simulink model "sstdr_basic"  (R2024b)
settings: Solver=FixedStepDiscrete  StartTime=0.0  StopTime=0.0005  FixedStep=5e-9  RelTol=1e-3
libraries: spsGroundLib x5, spsSeriesRLCBranchLib x4, spsIdealSwitchLib x3, spsVoltageMeasurementLib x3, spsControlledVoltageSourceLib x1, dspstat3 x1, spsDistributedParametersLineFrequencyDependentLib x1, sps_lib x1
settings Model: Creator=nathanielfargo  LastModifiedBy=nathanielfargo

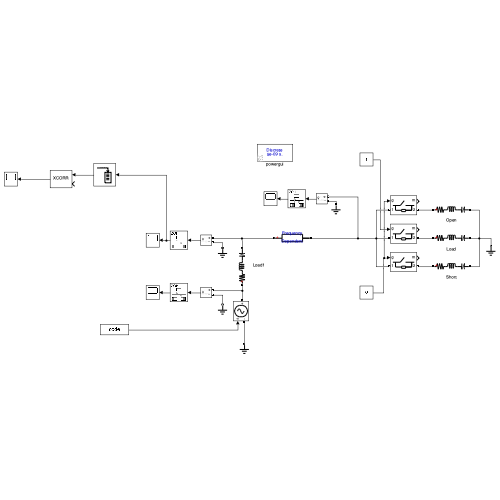
[thumbnail: Simulink's stored preview of the top-level diagram]
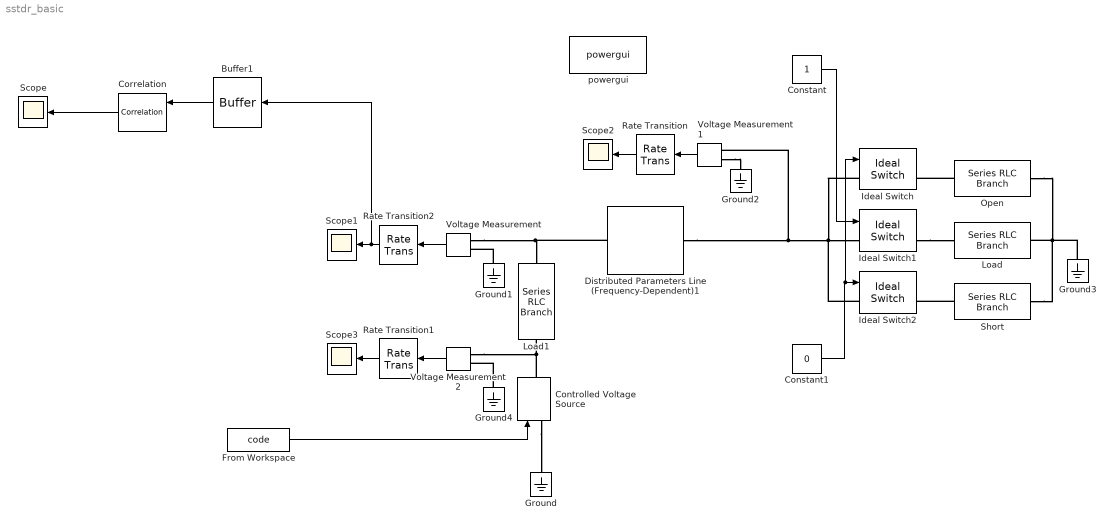
== system sstdr_basic ==
  Buffer1 : Buffer  N=100  V=99  OutputFrames=off
  Constant : Constant
  Constant1 : Constant  Value=0
  Controlled Voltage Source : spsControlledVoltageSourceLib/Controlled Voltage Source  Initialize=on  Source_Type=DC  Amplitude=0  Phase=0  Frequency=0  Measurements=None
  Correlation : dspstat3/Correlation  domain=Frequency  roundingMode=Floor  overflowMode=off  outputDataTypeStr=Inherit: Same as accumulator  outputMin=[]  outputMax=[]  outputLastDataTypeStr=Inherit: Same as accumulator
  Distributed Parameters Line (Frequency-Dependent)1 : spsDistributedParametersLineFrequencyDependentLib/Distributed Parameters Line (Frequency-Dependent)  WBfile=/Users/nathanielfargo/Desktop/school/Summer-25/wired/sstdr-simulation/simscape/line_test.mat  L=5  NbPhases=1  Frange=1.00e+00 Hz to 1.00e+05 Hz, 141 points.  Comments=|  Measurements=None
      | Example of a 735 KV three-phase line
      |
      | Three bundles of 4 Bersfort ACSR 1355 MCM conductors
      | Two 1/2 inch diameter steel grounds wires
      |
      | Ytower =Ymin =  average heights of conductors
      settings: LibrarySourceBlock=|
      | sps_lib/Power Grid Elements/Distributed Parameters Line
      | (Frequency-Dependent)
  From Workspace : FromWorkspace  VariableName=code  SampleTime=1/25e6
  Ground{,1..4} (5 alike) : spsGroundLib/Ground  LConnTagsString=a
  Ideal Switch : spsIdealSwitchLib/Ideal Switch  Ron=0.001  Lon=0  IC=1  Rs=1e5  Cs=inf  Measurements=on
  Ideal Switch1 : spsIdealSwitchLib/Ideal Switch  Ron=0.001  Lon=0  IC=0  Rs=1e5  Cs=inf  Measurements=on
  Ideal Switch2 : spsIdealSwitchLib/Ideal Switch  Ron=0.001  Lon=0  IC=0  Rs=1e5  Cs=inf  Measurements=on
  Load : spsSeriesRLCBranchLib/Series RLC Branch  LConnTagsString=__new0  RConnTagsString=__new0  BranchType=RLC  Resistance=50  Inductance=0  SetiL0=off  InitialCurrent=0  Capacitance=0  Setx0=off  InitialVoltage=0  Measurements=None
  Load1 : spsSeriesRLCBranchLib/Series RLC Branch  LConnTagsString=__new0  RConnTagsString=__new0  BranchType=RLC  Resistance=50  Inductance=0  SetiL0=off  InitialCurrent=0  Capacitance=1e-6  Setx0=off  InitialVoltage=0  Measurements=None
  Open : spsSeriesRLCBranchLib/Series RLC Branch  LConnTagsString=__new0  RConnTagsString=__new0  BranchType=RLC  Resistance=1e7  Inductance=0  SetiL0=off  InitialCurrent=0  Capacitance=0  Setx0=off  InitialVoltage=0  Measurements=None
  Rate Transition : RateTransition  OutPortSampleTime=1/50e6
  Rate Transition1 : RateTransition  OutPortSampleTime=1/50e6
  Rate Transition2 : RateTransition  OutPortSampleTime=1/50e6
  Scope{,1..3} (4 alike) : Scope
  Short : spsSeriesRLCBranchLib/Series RLC Branch  LConnTagsString=__new0  RConnTagsString=__new0  BranchType=RLC  Resistance=0  Inductance=0  SetiL0=off  InitialCurrent=0  Capacitance=0  Setx0=off  InitialVoltage=0  Measurements=None
  Voltage Measurement : spsVoltageMeasurementLib/Voltage Measurement  PhasorSimulation=off  OutputType=Complex  PSBequivalent=0
  Voltage Measurement1 : spsVoltageMeasurementLib/Voltage Measurement  PhasorSimulation=off  OutputType=Complex  PSBequivalent=0
  Voltage Measurement2 : spsVoltageMeasurementLib/Voltage Measurement  PhasorSimulation=off  OutputType=Complex  PSBequivalent=0
  powergui : sps_lib/powergui  Priority=1  SimulationMode=Discrete  SampleTime=5e-9  frequency=60  Iterations=50  frequencyindice=0  Pbase=100e6  ErrMax=1e-4  UnitsV=kV  UnitsW=MW  buscounter=0  FunctionMessages=off  echomessages=off  EnableUseOfTLC=off  CurrentSourceSwitches=off  DisableSnubberDevices=off  DisableRonSwitches=off  DisableVfSwitches=off  DisplayEquations=off  AutomaticDiscreteSolvers=off  SolverType=Tustin/Backward Euler (TBE)  Interpol=off  ExternalGateDelay=off  methode=off  Ts=100  x0status=blocks  SPID=on  SwTol=0  HookPort=off  NonlinearTolerance=1e-4  nMaxIteration=100  ContinueOnMaxIteration=off  RestoreLinks=warning  ResistiveCurrentMeasurement=off  Frange=[0:2:500]  Ylog=off  Xlog=on  ShowGrid=off  save=off  variable=ZData  structure=0  ZoomFFT=off  StartTime=0.0  cycles=1  DisplayStyle=1  fundamental=60  FreqAxis=off  MaxFrequency=1000  frequencyindicesteady=1  RmsSteady=1  display=off
  wires:
  From Workspace/1 -> Controlled Voltage Source/1
  Correlation/1 -> Scope/1
  Constant/1 -> Ideal Switch1/1
  Constant1/1 -> Ideal Switch/1, Ideal Switch2/1
  Buffer1/1 -> Correlation/1
  Voltage Measurement1/1 -> Rate Transition/1
  Rate Transition/1 -> Scope2/1
  Voltage Measurement2/1 -> Rate Transition1/1
  Rate Transition1/1 -> Scope3/1
  Voltage Measurement/1 -> Rate Transition2/1
  Rate Transition2/1 -> Scope1/1, Buffer1/1
  connections:
  Controlled Voltage Source/RConn1 -- Voltage Measurement2/LConn1 -- Load1/LConn1
  Controlled Voltage Source/LConn1 -- Ground/LConn1
  Ground1/LConn1 -- Voltage Measurement/LConn2
  Short/LConn1 -- Ideal Switch2/RConn1
  Ideal Switch1/RConn1 -- Load/LConn1
  Open/LConn1 -- Ideal Switch/RConn1
  Ideal Switch/LConn1 -- Voltage Measurement1/LConn1 -- Distributed Parameters Line (Frequency-Dependent)1/RConn1 -- Ideal Switch2/LConn1 -- Ideal Switch1/LConn1
  Voltage Measurement1/LConn2 -- Ground2/LConn1
  Ground3/LConn1 -- Open/RConn1 -- Short/RConn1 -- Load/RConn1
  Ground4/LConn1 -- Voltage Measurement2/LConn2
  Distributed Parameters Line (Frequency-Dependent)1/LConn1 -- Voltage Measurement/LConn1 -- Load1/RConn1
